simulink model "zhihoumoni"  (Simulink 7.4)
settings: Solver=ode45  StartTime=0.0  StopTime=2880  RelTol=1e-3
settings Model: Creator=admini  LastModifiedBy=admini

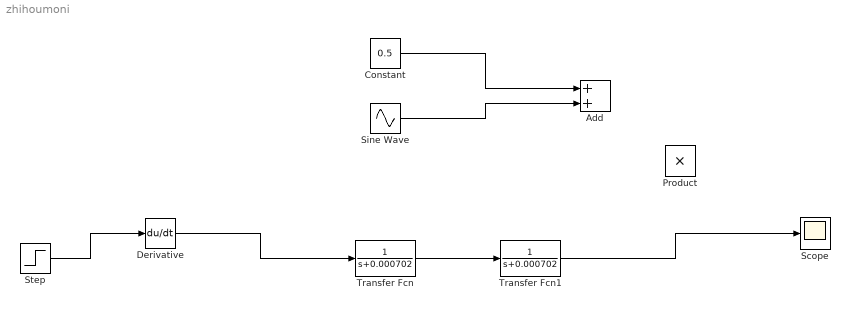
== system zhihoumoni ==
  Add : Sum  OutDataType=fixdt(1, 16)  OutScaling=2^-10
  Constant : Constant  Value=0.5  OutDataType=fixdt(1, 16)  OutScaling=2^0
  Derivative : Derivative
  Product : Product  OutDataType=fixdt(1, 16)  OutScaling=2^0  RndMeth=Zero
  Scope : Scope
  Sine Wave : Sin  Amplitude=0.5  Bias=0  Frequency=2*pi/1440  Phase=0  Samples=10  SampleTime=0  Offset=0
  Step : Step  After=53440  SampleTime=0
  Transfer Fcn : TransferFcn  Denominator=[1 0.000702]
  Transfer Fcn1 : TransferFcn  Denominator=[1 0.000702]
  wires:
  Step/1 -> Derivative/1
  Derivative/1 -> Transfer Fcn/1
  Transfer Fcn/1 -> Transfer Fcn1/1
  Constant/1 -> Add/1
  Sine Wave/1 -> Add/2
  Transfer Fcn1/1 -> Scope/1
